simulink model "fanghua"  (R2022b)
settings: Solver=FixedStepDiscrete  StartTime=0.0  StopTime=10.0  FixedStep=0.01  RelTol=1e-3
undefined symbols (not defined in the file): R, sigbuilder_block
libraries: simulink x10
settings Model: Creator=YJR  LastModifiedBy=YJR

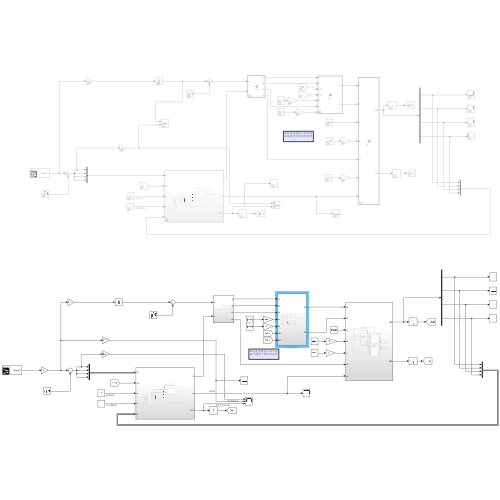
[thumbnail: Simulink's stored preview of the top-level diagram]
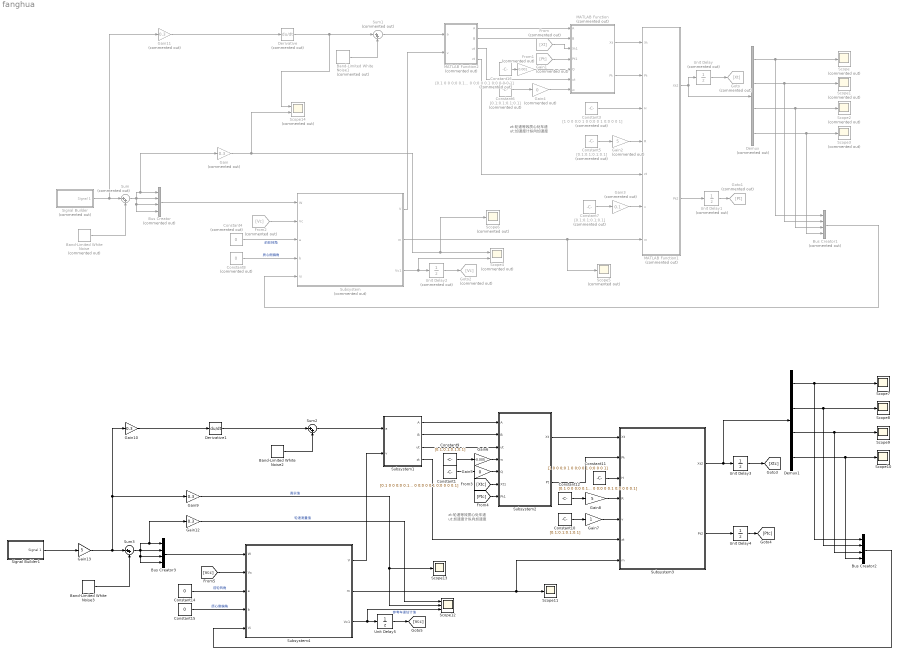
== system fanghua ==
  note: zt:轮速等效质心处车速
      | ut:加速度计纵向加速度
  note: zt:轮速等效质心处车速
      | ut:加速度计纵向加速度
  Band-Limited White Noise : simulink/Sources/Band-Limited White Noise  Commented=on  Cov=[0.05]  Ts=0.05  seed=[23341]
  Band-Limited White Noise1 : simulink/Sources/Band-Limited White Noise  Commented=on  Cov=[0.1]  Ts=0.1  seed=[23341]
  Band-Limited White Noise2 : simulink/Sources/Band-Limited White Noise  Cov=[0.1]  Ts=0.01  seed=[23341]
  Band-Limited White Noise3 : simulink/Sources/Band-Limited White Noise  Cov=[0.05]  Ts=0.01  seed=[23341]
  Bus Creator : BusCreator  Commented=on  Inputs=4
  Bus Creator1 : BusCreator  Commented=on  Inputs=4
  Bus Creator2 : BusCreator  Inputs=4
  Bus Creator3 : BusCreator  Inputs=4
  Constant1 : Constant  Value=[0.1 0 0 0;0 0.1 0 0;0 0 0.1 0;0 0 0 0.1]
  Constant10 : Constant  Value=[0.1;0.1;0.1;0.1]
  Constant11 : Constant  Value=[1 0 0 0;0 1 0 0;0 0 1 0;0 0 0 1]
  Constant12 : Constant  Value=[0.1 0 0 0;0 0.1 0 0;0 0 0.1 0;0 0 0 0.1]
  Constant14 : Constant  Value=0
  Constant15 : Constant  Value=0
  Constant16 : Constant  Commented=on  Value=[0.1 0 0 0;0 0.1 0 0;0 0 0.1 0;0 0 0 0.1]
  Constant3 : Constant  Commented=on  Value=[1 0 0 0;0 1 0 0;0 0 1 0;0 0 0 1]
  Constant4 : Constant  Commented=on  Value=0
  Constant5 : Constant  Commented=on  Value=[0.1;0.1;0.1;0.1]
  Constant6 : Constant  Commented=on  Value=[0.1;0.1;0.1;0.1]
  Constant7 : Constant  Commented=on  Value=[0.1;0.1;0.1;0.1]
  Constant8 : Constant  Commented=on  Value=0
  Constant9 : Constant  Value=[0.1;0.1;0.1;0.1]
  Demux : Demux  Commented=on
  Demux1 : Demux
  Derivative : Derivative  Commented=on
  Derivative1 : Derivative
  From : From  Commented=on  GotoTag=Xt
  From1 : From  Commented=on  GotoTag=Pt
  From2 : From  Commented=on  GotoTag=Vc
  Gain : Gain  Commented=on  Gain=0.3
  Gain1 : Gain  Commented=on  Gain=0.001
  Gain10 : Gain  Gain=0.3
  Gain11 : Gain  Commented=on  Gain=0.3
  Gain12 : Gain  Gain=0.3
  Gain13 : Gain  Gain=5
  Gain2 : Gain  Commented=on  Gain=5
  Gain3 : Gain  Commented=on  Gain=0.1
  Gain4 : Gain  Commented=on  Gain=0
  Gain5 : Gain  Gain=0
  Gain6 : Gain  Gain=-0.005
  Gain7 : Gain
  Gain8 : Gain  Gain=5
  Gain9 : Gain  Gain=0.3
  Goto : Goto  Commented=on  GotoTag=Xt
  Goto1 : Goto  Commented=on  GotoTag=Pt
  Goto2 : Goto  Commented=on  GotoTag=Vc
  MATLAB Function : MATLAB Function  Commented=on  TreatAsAtomicUnit=on
  MATLAB Function1 : MATLAB Function  Commented=on  TreatAsAtomicUnit=on
  MATLAB Function2 : MATLAB Function  Commented=on  TreatAsAtomicUnit=on
  Scope{,1..3,5..6} (6 alike) : Scope  Commented=on
  Scope{7..11,13} (6 alike) : Scope
  Scope12 : Scope  NumInputPorts=3
  Scope14 : Scope  Commented=on  NumInputPorts=2
  Scope4 : Scope  Commented=on  NumInputPorts=2
  Signal Builder : Subsystem  Tag=STV Subsys  Commented=on  LoadFcn=sigbuilder_block('load');  StartFcn=sigbuilder_block('start');  StopFcn=sigbuilder_block('stop');  ClipboardFcn=sigbuilder_block('clipboard');  mask(Sigbuilder block){tuvar=[0:10]}
      mask help: Simulink:masks:SigbuilderBlock_MD
      mask init:
      | if ~strcmp(get_param(bdroot(gcbh),'SimulationStatus'),'stopped') tuvar = sigbuilder_block('maskInit'); end
      settings: CopyFcn=sigbuilder_block('copy');  DeleteFcn=sigbuilder_block('delete');  ModelCloseFcn=sigbuilder_block('modelClose');  PreSaveFcn=sigbuilder_block('preSave');  PauseFcn=sigbuilder_block('pause');  ContinueFcn=sigbuilder_block('continue');  NameChangeFcn=sigbuilder_block('namechange');  OpenFcn=sigbuilder_block('open',[437.6 199.2 550.4 400 ]);  CloseFcn=sigbuilder_block('close');
      mask Display: plot(0, 0, 100, 100,[2, 2, 32, 32, 2], [68, 8, 8, 68, 68],[32, 2], [38, 38], [32, 19, 2],[53, 60, 44], [32, 17, 17, 2],[16, 16, 31, 31]);txt = getActiveGroup(gcbh);text(2, 100, txt,'verticalAlignment', 'top');
  Signal Builder1 : Subsystem  Tag=STV Subsys  LoadFcn=sigbuilder_block('load');  StartFcn=sigbuilder_block('start');  StopFcn=sigbuilder_block('stop');  ClipboardFcn=sigbuilder_block('clipboard');  mask(Sigbuilder block){tuvar=[0:10]}
      mask help: Simulink:masks:SigbuilderBlock_MD
      mask init:
      | if ~strcmp(get_param(bdroot(gcbh),'SimulationStatus'),'stopped') tuvar = sigbuilder_block('maskInit'); end
      settings: CopyFcn=sigbuilder_block('copy');  DeleteFcn=sigbuilder_block('delete');  ModelCloseFcn=sigbuilder_block('modelClose');  PreSaveFcn=sigbuilder_block('preSave');  PauseFcn=sigbuilder_block('pause');  ContinueFcn=sigbuilder_block('continue');  NameChangeFcn=sigbuilder_block('namechange');  OpenFcn=sigbuilder_block('open',[437.6 199.2 550.4 400 ]);  CloseFcn=sigbuilder_block('close');
      mask Display: plot(0, 0, 100, 100,[2, 2, 32, 32, 2], [68, 8, 8, 68, 68],[32, 2], [38, 38], [32, 19, 2],[53, 60, 44], [32, 17, 17, 2],[16, 16, 31, 31]);txt = getActiveGroup(gcbh);text(2, 100, txt,'verticalAlignment', 'top');
  Subsystem : Subsystem  Commented=on
  Subsystem1 : Subsystem
  Subsystem2 : Subsystem
  Subsystem3 : Subsystem
  Subsystem4 : Subsystem
  Sum : Sum  Commented=on  Inputs=|++
  Sum1 : Sum  Commented=on  Inputs=|++
  Sum2 : Sum  Inputs=|++
  Sum3 : Sum  Inputs=|++
  Unit Delay : UnitDelay  Commented=on  SampleTime=-1  HasFrameUpgradeWarning=on
  Unit Delay1 : UnitDelay  Commented=on  SampleTime=-1  HasFrameUpgradeWarning=on
  Unit Delay2 : UnitDelay  Commented=on  SampleTime=-1  HasFrameUpgradeWarning=on
  Unit Delay3 : UnitDelay  SampleTime=-1  HasFrameUpgradeWarning=on
  Unit Delay4 : UnitDelay  SampleTime=-1  HasFrameUpgradeWarning=on
  Unit Delay5 : UnitDelay  SampleTime=-1  HasFrameUpgradeWarning=on
  wires:
  MATLAB Function1/2(Pt2) -> Unit Delay1/1
  MATLAB Function/1(Xt) -> MATLAB Function1/1(Xt)
  MATLAB Function/2(Pt) -> MATLAB Function1/2(Pt)
  MATLAB Function2/1(A) -> MATLAB Function/1(A)
  MATLAB Function2/2(B) -> MATLAB Function/2(B)
  Constant16/1 -> Gain1/1
  Constant3/1 -> MATLAB Function1/3(H)
  MATLAB Function2/3(ut) -> MATLAB Function/6(ut)
  Demux/1 -> Bus Creator1/1, Scope/1
  Demux/2 -> Bus Creator1/2, Scope1/1
  Constant5/1 -> Gain2/1
  MATLAB Function2/4(zt) -> MATLAB Function1/5(zt)
  Constant6/1 -> Gain4/1
  From/1 -> MATLAB Function/3(Xt1)
  Unit Delay/1 -> Goto/1
  From1/1 -> MATLAB Function/4(Pt1)
  Unit Delay1/1 -> Goto1/1
  Constant7/1 -> Gain3/1
  Demux/3 -> Bus Creator1/3, Scope2/1
  Demux/4 -> Bus Creator1/4, Scope3/1
  Subsystem/2(m) -> Scope5/1, MATLAB Function1/7(m)
  Gain1/1 -> MATLAB Function/5(Q)
  Gain2/1 -> MATLAB Function1/4(R)
  Gain3/1 -> MATLAB Function1/6(v)
  Subsystem/1(V) -> MATLAB Function2/2(v)
  Subsystem/3(Vc1) -> Scope4/2, Unit Delay2/1
  From2/1 -> Subsystem/2(Vc)
  Unit Delay2/1 -> Goto2/1
  MATLAB Function1/1(Xt2) -> Unit Delay/1, Demux/1
  Bus Creator1/1 -> Subsystem/5(Vi)
  Constant4/1 -> Subsystem/3(a)  "前轮转角"
  Constant8/1 -> Subsystem/4(b)  "质心侧偏角"
  Bus Creator/1 -> Subsystem/1(W)
  Sum/1 -> Gain/1, Bus Creator/1, Bus Creator/2, Bus Creator/3, Bus Creator/4
  Gain/1 -> Scope14/2, Scope6/1, Scope4/1
  Band-Limited White Noise/1 -> Sum/2
  Sum1/1 -> MATLAB Function2/1(a)
  Gain4/1 -> MATLAB Function/7(w)
  Derivative/1 -> Scope14/1, Sum1/1
  Band-Limited White Noise1/1 -> Sum1/2
  Subsystem1/1(A) -> Subsystem2/1(A)
  Subsystem1/2(B) -> Subsystem2/2(B)
  Subsystem1/3(ut) -> Subsystem2/3(ut)
  Gain5/1 -> Subsystem2/5(Q)
  Constant1/1 -> Gain5/1
  Constant9/1 -> Gain6/1
  Gain6/1 -> Subsystem2/4(w)
  [Xtc] -> Subsystem2/6(Xt1)
  [Ptc] -> Subsystem2/7(Pt1)
  Constant10/1 -> Gain7/1
  Gain7/1 -> Subsystem3/5(v)
  Subsystem1/4(zt) -> Subsystem3/6(zt)
  Subsystem2/1(Xt) -> Subsystem3/1(Xt)
  Subsystem2/2(Pt) -> Subsystem3/2(Pt)
  Constant11/1 -> Subsystem3/3(H)
  Constant12/1 -> Gain8/1
  Gain8/1 -> Subsystem3/4(R)
  Subsystem3/1(Xt2) -> Demux1/1, Unit Delay3/1
  Unit Delay3/1 -> [Xtc]
  Unit Delay4/1 -> [Ptc]
  Subsystem3/2(Pt2) -> Unit Delay4/1
  Band-Limited White Noise2/1 -> Sum2/2
  Derivative1/1 -> Sum2/1
  Sum2/1 -> Subsystem1/1(a)
  Demux1/4 -> Scope10/1, Bus Creator2/4
  Demux1/3 -> Scope9/1, Bus Creator2/3
  Demux1/2 -> Scope8/1, Bus Creator2/2
  Demux1/1 -> Scope7/1, Bus Creator2/1
  Band-Limited White Noise3/1 -> Sum3/2
  Gain9/1 -> Scope12/2, Scope13/1  "真实值"
  Sum3/1 -> Bus Creator3/4, Bus Creator3/3, Bus Creator3/2, Gain12/1, Bus Creator3/1
  Bus Creator3/1 -> Subsystem4/1(W)
  Constant15/1 -> Subsystem4/4(b)  "质心侧偏角"
  Constant14/1 -> Subsystem4/3(a)  "前轮转角"
  Bus Creator2/1 -> Subsystem4/5(Vi)
  Signal Builder1/1(Signal 1) -> Gain13/1
  Unit Delay5/1 -> [Vcc]
  [Vcc] -> Subsystem4/2(Vc)
  Subsystem4/3(Vc1) -> Scope12/3, Unit Delay5/1  "参考车速估计值"
  Subsystem4/1(V) -> Subsystem1/2(v)
  Subsystem4/2(m) -> Scope11/1, Subsystem3/7(m)
  Signal Builder/1(Signal 1) -> Gain11/1, Sum/1
  Gain10/1 -> Derivative1/1
  Gain11/1 -> Derivative/1
  Gain12/1 -> Scope12/1  "轮速测量值"
  Gain13/1 -> Gain9/1, Gain10/1, Sum3/1

== system fanghua/Signal Builder ==
  Demux : Demux  Tag=STV Demux  Outputs=1
      settings: DisplayOption=none
  FromWs : FromWorkspace  Tag=STV FromWs  VariableName=tuvar
      SigBuilderData=|
      | common.afterFinalStr = 'Extrapolate'
      | common.sampleTime = 0
      | dataSet.timeRange = [0 10]
      | dataSet.name = 'Group 1'
      | sbobj.Groups.Name = 'Group 1'
      | sbobj.Groups.Signals.Name = 'Signal 1'
      | sbobj.Groups.Signals.XData = [0 3 4 6 8 10]
      | sbobj.Groups.Signals.YData = [0 6.8 30 26.4 0 0]
  Signal 1 : Outport  Tag=STV Outport
  wires:
  FromWs/1 -> Demux/1
  Demux/1 -> Signal 1/1

== system fanghua/Signal Builder1 ==
  Demux : Demux  Tag=STV Demux  Outputs=1
      settings: DisplayOption=none
  FromWs : FromWorkspace  Tag=STV FromWs  VariableName=tuvar
      SigBuilderData=|
      | common.afterFinalStr = 'Extrapolate'
      | common.sampleTime = 0
      | dataSet.timeRange = [0 10]
      | dataSet.name = 'Group 1'
      | sbobj.Groups.Name = 'Group 1'
      | sbobj.Groups.Signals.Name = 'Signal 1'
      | sbobj.Groups.Signals.XData = [0 3 4 6 8 10]
      | sbobj.Groups.Signals.YData = [0 6.8 30 22 36 0]
  Signal 1 : Outport  Tag=STV Outport
  wires:
  Demux/1 -> Signal 1/1
  FromWs/1 -> Demux/1

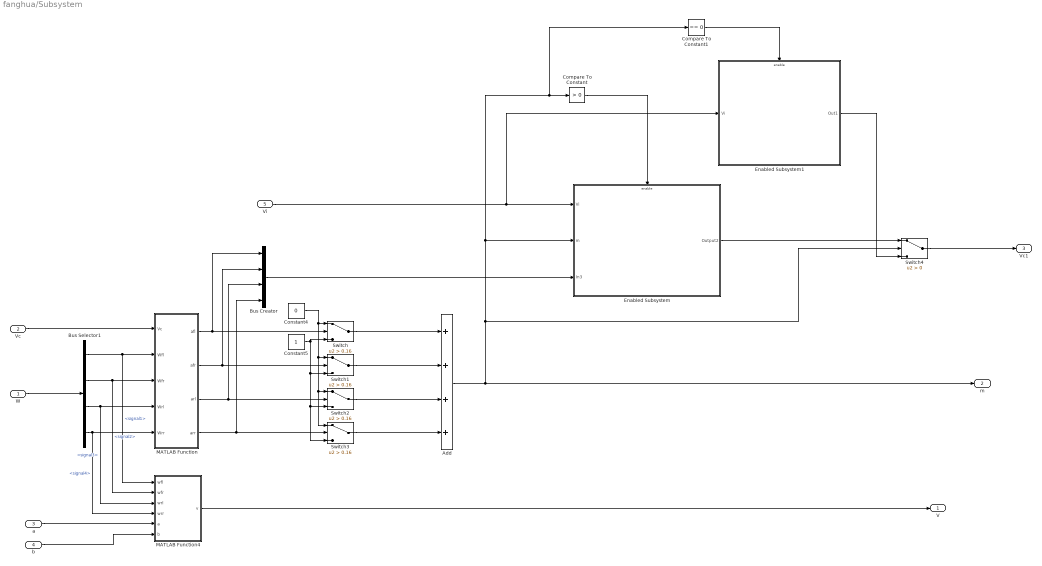
== system fanghua/Subsystem ==
  W : Inport
  Vc : Inport  Port=2
  a : Inport  Port=3
  b : Inport  Port=4
  Vi : Inport  Port=5
  Add : Sum  Inputs=++++
  Bus Creator : BusCreator  Inputs=4
  Bus Selector1 : BusSelector  OutputSignals=signal1,signal2,signal3,signal4
  Compare To Constant : simulink/Logic and Bit Operations/Compare To Constant  relop=>  const=0  OutDataTypeStr=boolean
  Compare To Constant1 : simulink/Logic and Bit Operations/Compare To Constant  relop===  const=0  OutDataTypeStr=boolean
  Constant4 : Constant  Value=0
  Constant5 : Constant
  Enabled Subsystem : Subsystem  TreatAsAtomicUnit=on
  Enabled Subsystem1 : Subsystem  TreatAsAtomicUnit=on
  MATLAB Function : MATLAB Function  TreatAsAtomicUnit=on
  MATLAB Function4 : MATLAB Function  TreatAsAtomicUnit=on
  Switch{,1..3} (4 alike) : Switch  Criteria=u2 > Threshold  Threshold=0.16  SaturateOnIntegerOverflow=off  InputSameDT=off
  Switch4 : Switch  Criteria=u2 > Threshold  SaturateOnIntegerOverflow=off  InputSameDT=off
  V : Outport
  m : Outport  Port=2
  Vc1 : Outport  Port=3
  wires:
  Constant5/1 -> Switch3/3, Switch2/3, Switch1/3, Switch/3
  Constant4/1 -> Switch3/1, Switch2/1, Switch1/1, Switch/1
  Add/1 -> Switch4/2, Enabled Subsystem/2(m), Compare To Constant1/1, Compare To Constant/1, m/1
  Bus Selector1/1 -> MATLAB Function4/1(wfl), MATLAB Function/2(Wfl)  "<signal1>"
  Bus Selector1/2 -> MATLAB Function4/2(wfr), MATLAB Function/3(Wfr)  "<signal2>"
  Bus Selector1/3 -> MATLAB Function4/3(wrl), MATLAB Function/4(Wrl)  "<signal3>"
  Bus Selector1/4 -> MATLAB Function4/4(wrr), MATLAB Function/5(Wrr)  "<signal4>"
  W/1 -> Bus Selector1/1
  MATLAB Function/1(afl) -> Bus Creator/1, Switch/2
  MATLAB Function/2(afr) -> Bus Creator/2, Switch1/2
  MATLAB Function/3(arl) -> Bus Creator/3, Switch2/2
  MATLAB Function/4(arr) -> Bus Creator/4, Switch3/2
  Vc/1 -> MATLAB Function/1(Vc)
  MATLAB Function4/1(v) -> V/1
  Switch/1 -> Add/1
  Switch3/1 -> Add/4
  Switch2/1 -> Add/3
  Switch1/1 -> Add/2
  a/1 -> MATLAB Function4/5(a)
  b/1 -> MATLAB Function4/6(b)
  Vi/1 -> Enabled Subsystem1/1(Vi), Enabled Subsystem/1(Vi)
  Compare To Constant/1 -> Enabled Subsystem/Enable
  Bus Creator/1 -> Enabled Subsystem/3(In3)
  Compare To Constant1/1 -> Enabled Subsystem1/Enable
  Enabled Subsystem/1(Output2) -> Switch4/1
  Enabled Subsystem1/1(Out1) -> Switch4/3
  Switch4/1 -> Vc1/1

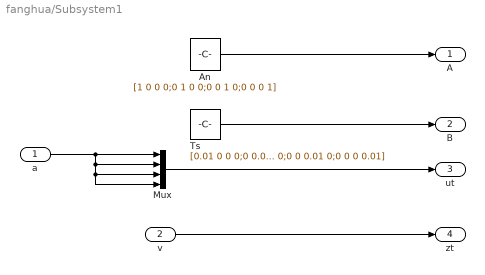
== system fanghua/Subsystem1 ==
  a : Inport
  v : Inport  Port=2
  An : Constant  Value=[1 0 0 0;0 1 0 0;0 0 1 0;0 0 0 1]
  Mux : Mux
  Ts : Constant  Value=[0.01 0 0 0;0 0.01 0 0;0 0 0.01 0;0 0 0 0.01]
  A : Outport
  B : Outport  Port=2
  ut : Outport  Port=3
  zt : Outport  Port=4
  wires:
  v/1 -> zt/1
  Mux/1 -> ut/1
  a/1 -> Mux/1, Mux/4, Mux/3, Mux/2
  An/1 -> A/1
  Ts/1 -> B/1

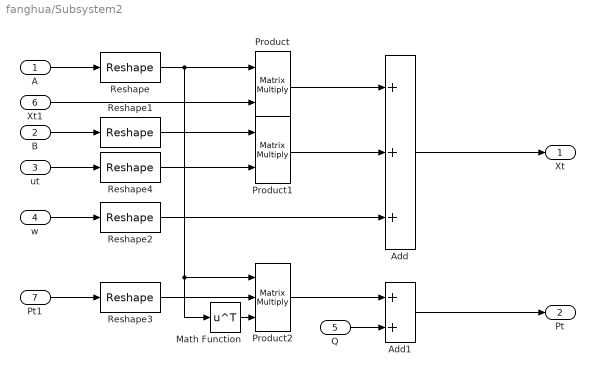
== system fanghua/Subsystem2 ==
  A : Inport
  B : Inport  Port=2
  ut : Inport  Port=3
  w : Inport  Port=4
  Q : Inport  Port=5
  Xt1 : Inport  Port=6
  Pt1 : Inport  Port=7
  Add : Sum  Inputs=+++
  Add1 : Sum
  Math Function : Math  Operator=transpose
  Product : Product  Multiplication=Matrix(*)
  Product1 : Product  Multiplication=Matrix(*)
  Product2 : Product  Inputs=3  Multiplication=Matrix(*)
  Reshape : Reshape  OutputDimensionality=Customize  OutputDimensions=[4,4]
  Reshape1 : Reshape  OutputDimensionality=Customize  OutputDimensions=[4,4]
  Reshape2 : Reshape  OutputDimensionality=Customize  OutputDimensions=[4,1]
  Reshape3 : Reshape  OutputDimensionality=Customize  OutputDimensions=[4,4]
  Reshape4 : Reshape  OutputDimensionality=Customize  OutputDimensions=[4,1]
  Xt : Outport
  Pt : Outport  Port=2
  wires:
  A/1 -> Reshape/1
  B/1 -> Reshape1/1
  Reshape/1 -> Math Function/1, Product2/1, Product/1
  Product/1 -> Add/1
  Xt1/1 -> Product/2
  Reshape1/1 -> Product1/1
  ut/1 -> Reshape4/1
  w/1 -> Reshape2/1
  Product1/1 -> Add/2
  Reshape2/1 -> Add/3
  Add/1 -> Xt/1
  Pt1/1 -> Reshape3/1
  Math Function/1 -> Product2/3
  Product2/1 -> Add1/1
  Q/1 -> Add1/2
  Add1/1 -> Pt/1
  Reshape3/1 -> Product2/2
  Reshape4/1 -> Product1/2

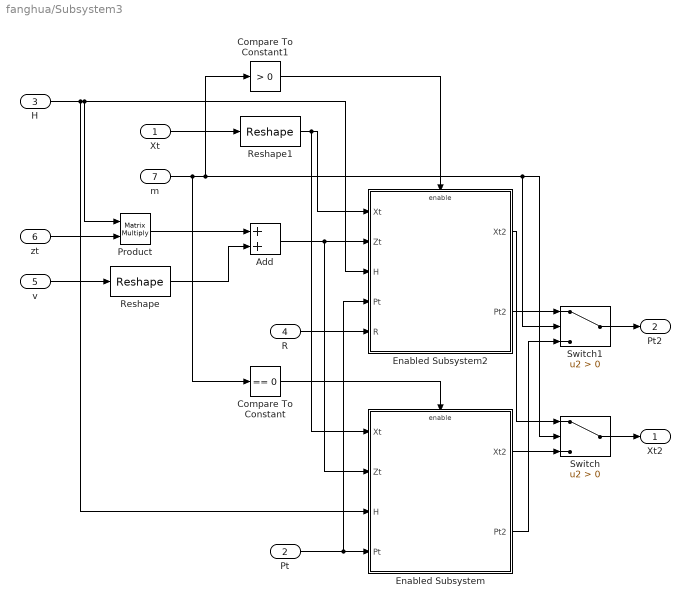
== system fanghua/Subsystem3 ==
  Xt : Inport
  Pt : Inport  Port=2
  H : Inport  Port=3
  R : Inport  Port=4
  v : Inport  Port=5
  zt : Inport  Port=6
  m : Inport  Port=7
  Add : Sum
  Compare To Constant : simulink/Logic and Bit Operations/Compare To Constant  relop===  const=0  OutDataTypeStr=boolean
  Compare To Constant1 : simulink/Logic and Bit Operations/Compare To Constant  relop=>  const=0  OutDataTypeStr=boolean
  Enabled Subsystem : Subsystem  TreatAsAtomicUnit=on
  Enabled Subsystem2 : Subsystem  TreatAsAtomicUnit=on
  Product : Product  Multiplication=Matrix(*)
  Reshape : Reshape  OutputDimensionality=Customize  OutputDimensions=[4,1]
  Reshape1 : Reshape  OutputDimensionality=Customize  OutputDimensions=[4,1]
  Switch : Switch  Criteria=u2 > Threshold  SaturateOnIntegerOverflow=off  InputSameDT=off
  Switch1 : Switch  Criteria=u2 > Threshold  SaturateOnIntegerOverflow=off  InputSameDT=off
  Xt2 : Outport
  Pt2 : Outport  Port=2
  wires:
  H/1 -> Enabled Subsystem2/3(H), Product/1, Enabled Subsystem/3(H)
  Switch/1 -> Xt2/1
  Compare To Constant1/1 -> Enabled Subsystem2/Enable
  zt/1 -> Product/2
  Enabled Subsystem/1(Xt2) -> Switch/3
  Reshape/1 -> Add/2
  Compare To Constant/1 -> Enabled Subsystem/Enable
  v/1 -> Reshape/1
  Product/1 -> Add/1
  m/1 -> Switch1/2, Switch/2, Compare To Constant1/1, Compare To Constant/1
  Xt/1 -> Reshape1/1
  Reshape1/1 -> Enabled Subsystem2/1(Xt), Enabled Subsystem/1(Xt)
  Add/1 -> Enabled Subsystem/2(Zt), Enabled Subsystem2/2(Zt)
  R/1 -> Enabled Subsystem2/5(R)
  Pt/1 -> Enabled Subsystem/4(Pt), Enabled Subsystem2/4(Pt)
  Enabled Subsystem2/1(Xt2) -> Switch/1
  Enabled Subsystem2/2(Pt2) -> Switch1/1
  Enabled Subsystem/2(Pt2) -> Switch1/3
  Switch1/1 -> Pt2/1

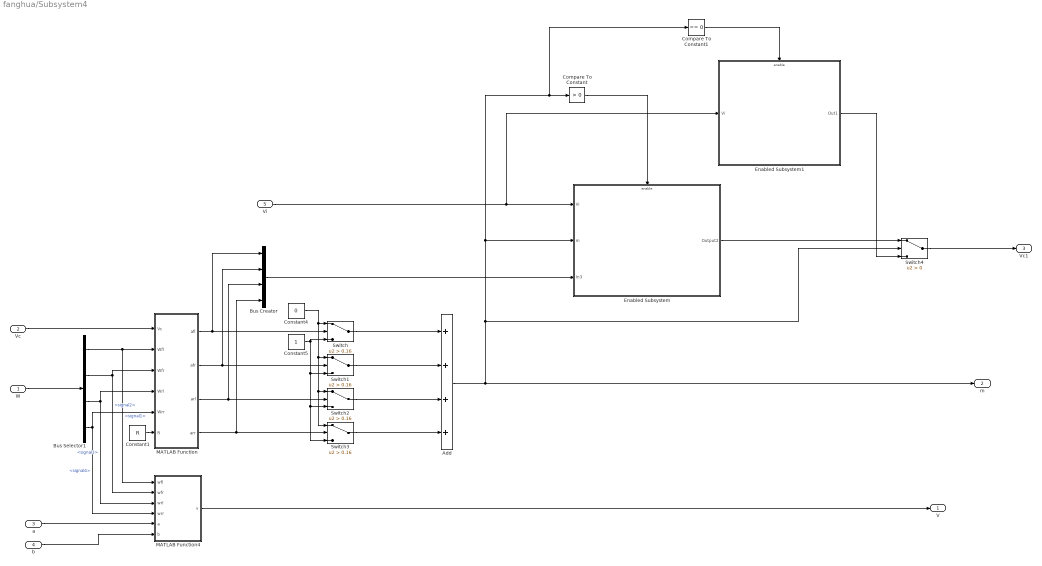
== system fanghua/Subsystem4 ==
  W : Inport
  Vc : Inport  Port=2
  a : Inport  Port=3
  b : Inport  Port=4
  Vi : Inport  Port=5
  Add : Sum  Inputs=++++
  Bus Creator : BusCreator  Inputs=4
  Bus Selector1 : BusSelector  OutputSignals=signal1,signal2,signal3,signal4
  Compare To Constant : simulink/Logic and Bit Operations/Compare To Constant  relop=>  const=0  OutDataTypeStr=boolean
  Compare To Constant1 : simulink/Logic and Bit Operations/Compare To Constant  relop===  const=0  OutDataTypeStr=boolean
  Constant1 : Constant  Value=R
  Constant4 : Constant  Value=0
  Constant5 : Constant
  Enabled Subsystem : Subsystem  TreatAsAtomicUnit=on
  Enabled Subsystem1 : Subsystem  TreatAsAtomicUnit=on
  MATLAB Function : MATLAB Function  TreatAsAtomicUnit=on
  MATLAB Function4 : MATLAB Function  TreatAsAtomicUnit=on
  Switch{,1..3} (4 alike) : Switch  Criteria=u2 > Threshold  Threshold=0.16  SaturateOnIntegerOverflow=off  InputSameDT=off
  Switch4 : Switch  Criteria=u2 > Threshold  SaturateOnIntegerOverflow=off  InputSameDT=off
  V : Outport
  m : Outport  Port=2
  Vc1 : Outport  Port=3
  wires:
  Switch4/1 -> Vc1/1
  Enabled Subsystem1/1(Out1) -> Switch4/3
  Enabled Subsystem/1(Output2) -> Switch4/1
  Compare To Constant1/1 -> Enabled Subsystem1/Enable
  Bus Creator/1 -> Enabled Subsystem/3(In3)
  Compare To Constant/1 -> Enabled Subsystem/Enable
  Vi/1 -> Enabled Subsystem/1(Vi), Enabled Subsystem1/1(Vi)
  b/1 -> MATLAB Function4/6(b)
  a/1 -> MATLAB Function4/5(a)
  Switch1/1 -> Add/2
  Switch2/1 -> Add/3
  Switch3/1 -> Add/4
  Switch/1 -> Add/1
  MATLAB Function4/1(v) -> V/1
  Vc/1 -> MATLAB Function/1(Vc)
  MATLAB Function/4(arr) -> Switch3/2, Bus Creator/4
  MATLAB Function/3(arl) -> Switch2/2, Bus Creator/3
  MATLAB Function/2(afr) -> Switch1/2, Bus Creator/2
  MATLAB Function/1(afl) -> Switch/2, Bus Creator/1
  W/1 -> Bus Selector1/1
  Bus Selector1/4 -> MATLAB Function4/4(wrr), MATLAB Function/5(Wrr)  "<signal4>"
  Bus Selector1/3 -> MATLAB Function4/3(wrl), MATLAB Function/4(Wrl)  "<signal3>"
  Bus Selector1/2 -> MATLAB Function4/2(wfr), MATLAB Function/3(Wfr)  "<signal2>"
  Bus Selector1/1 -> MATLAB Function4/1(wfl), MATLAB Function/2(Wfl)  "<signal1>"
  Add/1 -> m/1, Compare To Constant/1, Compare To Constant1/1, Enabled Subsystem/2(m), Switch4/2
  Constant4/1 -> Switch/1, Switch1/1, Switch2/1, Switch3/1
  Constant5/1 -> Switch/3, Switch1/3, Switch2/3, Switch3/3
  Constant1/1 -> MATLAB Function/6(R)

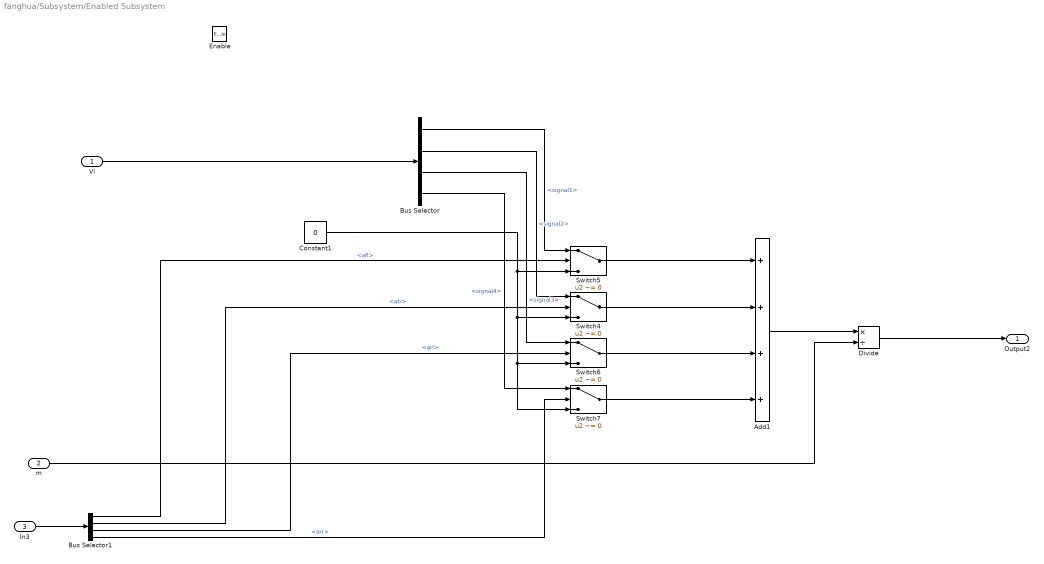
== system fanghua/Subsystem/Enabled Subsystem ==
  Vi : Inport
  m : Inport  Port=2
  In3 : Inport  Port=3
  Enable : EnablePort
  Add1 : Sum  Inputs=++++
  Bus Selector : BusSelector  OutputSignals=signal1,signal2,signal3,signal4
  Bus Selector1 : BusSelector  OutputSignals=afl,afr,arl,arr
  Constant1 : Constant  Value=0
  Divide : Product  Inputs=*/
  Switch{4..7} (4 alike) : Switch  Criteria=u2 ~= 0  Threshold=1  SaturateOnIntegerOverflow=off  InputSameDT=off
  Output2 : Outport
  wires:
  Bus Selector1/3 -> Switch6/2  "<arl>"
  Switch4/1 -> Add1/2
  Bus Selector1/2 -> Switch4/2  "<afr>"
  Bus Selector/3 -> Switch6/1  "<signal3>"
  Bus Selector/2 -> Switch4/1  "<signal2>"
  Constant1/1 -> Switch6/3, Switch7/3, Switch4/3, Switch5/3
  Bus Selector/1 -> Switch5/1  "<signal1>"
  m/1 -> Divide/2
  Bus Selector1/4 -> Switch7/2  "<arr>"
  Switch7/1 -> Add1/4
  Vi/1 -> Bus Selector/1
  Bus Selector/4 -> Switch7/1  "<signal4>"
  Switch6/1 -> Add1/3
  Add1/1 -> Divide/1
  Divide/1 -> Output2/1
  Switch5/1 -> Add1/1
  Bus Selector1/1 -> Switch5/2  "<afl>"
  In3/1 -> Bus Selector1/1

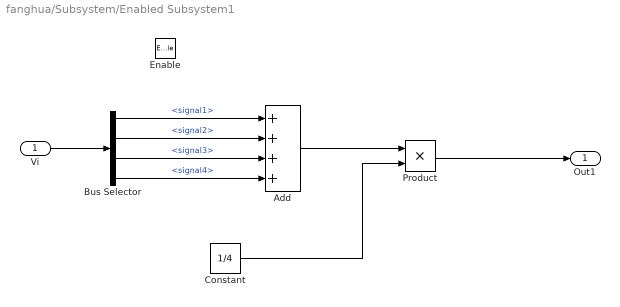
== system fanghua/Subsystem/Enabled Subsystem1 ==
  Vi : Inport
  Enable : EnablePort
  Add : Sum  Inputs=++++
  Bus Selector : BusSelector  OutputSignals=signal1,signal2,signal3,signal4
  Constant : Constant  Value=1/4
  Product : Product
  Out1 : Outport
  wires:
  Vi/1 -> Bus Selector/1
  Bus Selector/1 -> Add/1  "<signal1>"
  Bus Selector/3 -> Add/3  "<signal3>"
  Bus Selector/2 -> Add/2  "<signal2>"
  Bus Selector/4 -> Add/4  "<signal4>"
  Constant/1 -> Product/2
  Add/1 -> Product/1
  Product/1 -> Out1/1

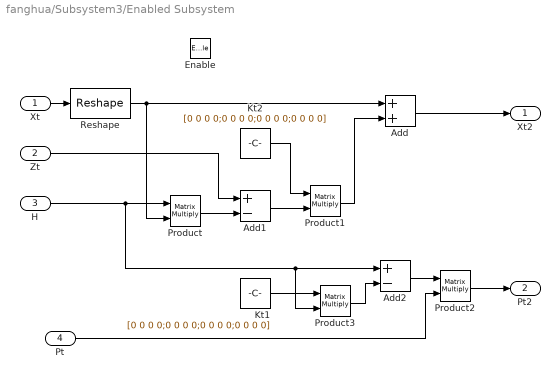
== system fanghua/Subsystem3/Enabled Subsystem ==
  Xt : Inport
  Zt : Inport  Port=2
  H : Inport  Port=3
  Pt : Inport  Port=4
  Enable : EnablePort
  Add : Sum
  Add1 : Sum  Inputs=+-
  Add2 : Sum  Inputs=+-
  Kt1 : Constant  Value=[0 0 0 0;0 0 0 0;0 0 0 0;0 0 0 0]
  Kt2 : Constant  Value=[0 0 0 0;0 0 0 0;0 0 0 0;0 0 0 0]
  Product{,1..3} (4 alike) : Product  Multiplication=Matrix(*)
  Reshape : Reshape  OutputDimensionality=Customize  OutputDimensions=[4,1]
  Xt2 : Outport
  Pt2 : Outport  Port=2
  wires:
  Xt/1 -> Reshape/1
  Add/1 -> Xt2/1
  Product/1 -> Add1/2
  Zt/1 -> Add1/1
  Add1/1 -> Product1/2
  Product1/1 -> Add/2
  H/1 -> Product3/2, Add2/1, Product/1
  Product3/1 -> Add2/2
  Add2/1 -> Product2/1
  Pt/1 -> Product2/2
  Product2/1 -> Pt2/1
  Kt1/1 -> Product3/1
  Reshape/1 -> Product/2, Add/1
  Kt2/1 -> Product1/1

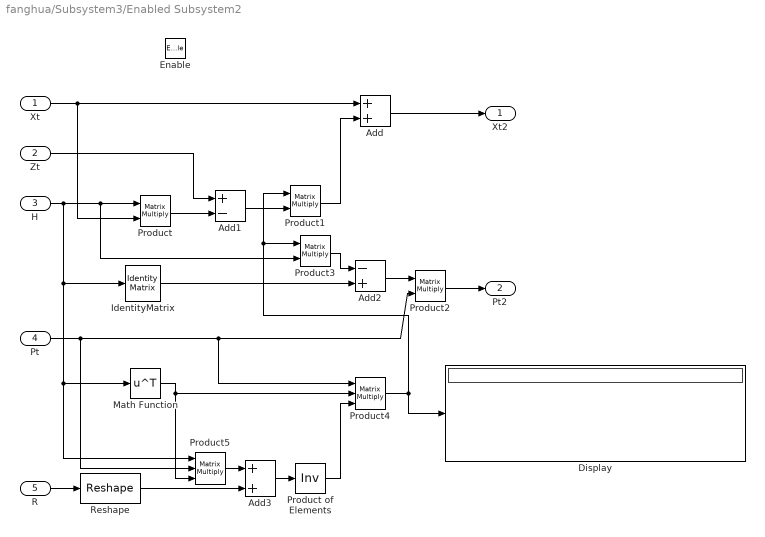
== system fanghua/Subsystem3/Enabled Subsystem2 ==
  Xt : Inport
  Zt : Inport  Port=2
  H : Inport  Port=3
  Pt : Inport  Port=4
  R : Inport  Port=5
  Enable : EnablePort
  Add : Sum
  Add1 : Sum  Inputs=+-
  Add2 : Sum  Inputs=-+
  Add3 : Sum
  Display : Display
  IdentityMatrix : IdentityMatrix  InheritOutputPortAttributes=on
  Math Function : Math  Operator=transpose
  Product{,1..3} (4 alike) : Product  Multiplication=Matrix(*)
  Product of Elements : Product  Inputs=/  Multiplication=Matrix(*)
  Product4 : Product  Inputs=3  Multiplication=Matrix(*)
  Product5 : Product  Inputs=3  Multiplication=Matrix(*)
  Reshape : Reshape  OutputDimensionality=Customize  OutputDimensions=[4,4]
  Xt2 : Outport
  Pt2 : Outport  Port=2
  wires:
  Product2/1 -> Pt2/1
  Pt/1 -> Product5/2, Product4/1, Product2/2
  Add2/1 -> Product2/1
  Product3/1 -> Add2/1
  IdentityMatrix/1 -> Add2/2
  Product1/1 -> Add/2
  Product4/1 -> Product1/1, Product3/1, Display/1
  Add1/1 -> Product1/2
  Zt/1 -> Add1/1
  Product/1 -> Add1/2
  H/1 -> Product/1, Product3/2, Product5/1, Math Function/1, IdentityMatrix/1
  Add/1 -> Xt2/1
  Xt/1 -> Add/1, Product/2
  Math Function/1 -> Product5/3, Product4/2
  Product5/1 -> Add3/1
  R/1 -> Reshape/1
  Add3/1 -> Product of Elements/1
  Product of Elements/1 -> Product4/3
  Reshape/1 -> Add3/2

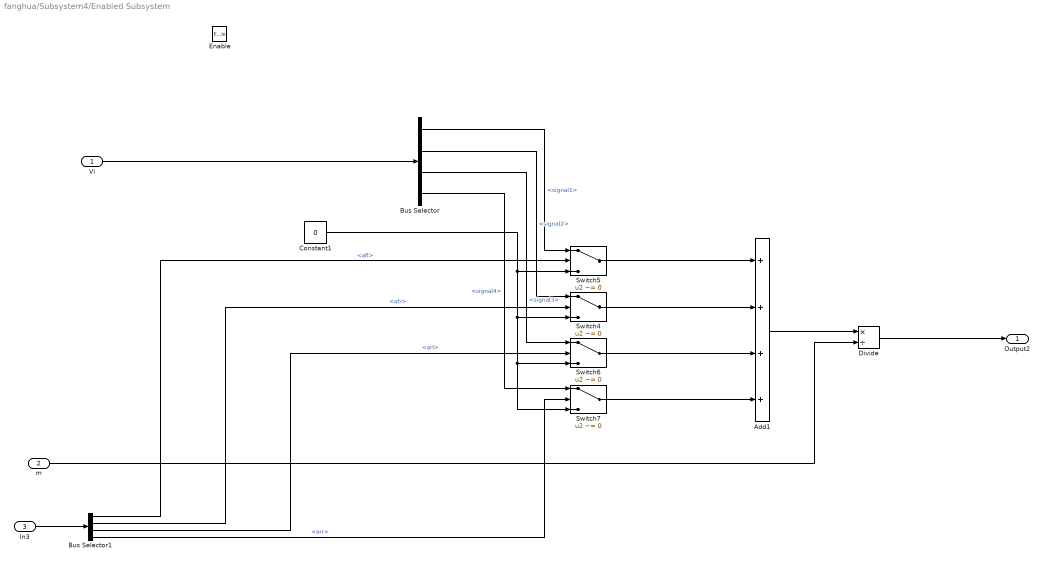
== system fanghua/Subsystem4/Enabled Subsystem ==
  Vi : Inport
  m : Inport  Port=2
  In3 : Inport  Port=3
  Enable : EnablePort
  Add1 : Sum  Inputs=++++
  Bus Selector : BusSelector  OutputSignals=signal1,signal2,signal3,signal4
  Bus Selector1 : BusSelector  OutputSignals=afl,afr,arl,arr
  Constant1 : Constant  Value=0
  Divide : Product  Inputs=*/
  Switch{4..7} (4 alike) : Switch  Criteria=u2 ~= 0  Threshold=1  SaturateOnIntegerOverflow=off  InputSameDT=off
  Output2 : Outport
  wires:
  In3/1 -> Bus Selector1/1
  Bus Selector1/1 -> Switch5/2  "<afl>"
  Switch5/1 -> Add1/1
  Divide/1 -> Output2/1
  Add1/1 -> Divide/1
  Switch6/1 -> Add1/3
  Bus Selector/4 -> Switch7/1  "<signal4>"
  Vi/1 -> Bus Selector/1
  Switch7/1 -> Add1/4
  Bus Selector1/4 -> Switch7/2  "<arr>"
  m/1 -> Divide/2
  Bus Selector/1 -> Switch5/1  "<signal1>"
  Constant1/1 -> Switch5/3, Switch4/3, Switch7/3, Switch6/3
  Bus Selector/2 -> Switch4/1  "<signal2>"
  Bus Selector/3 -> Switch6/1  "<signal3>"
  Bus Selector1/2 -> Switch4/2  "<afr>"
  Switch4/1 -> Add1/2
  Bus Selector1/3 -> Switch6/2  "<arl>"

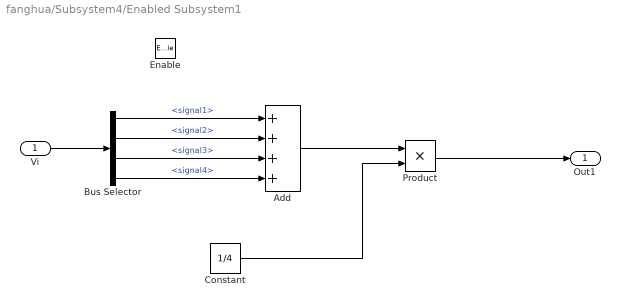
== system fanghua/Subsystem4/Enabled Subsystem1 ==
  Vi : Inport
  Enable : EnablePort
  Add : Sum  Inputs=++++
  Bus Selector : BusSelector  OutputSignals=signal1,signal2,signal3,signal4
  Constant : Constant  Value=1/4
  Product : Product
  Out1 : Outport
  wires:
  Product/1 -> Out1/1
  Add/1 -> Product/1
  Constant/1 -> Product/2
  Bus Selector/4 -> Add/4  "<signal4>"
  Bus Selector/2 -> Add/2  "<signal2>"
  Bus Selector/3 -> Add/3  "<signal3>"
  Bus Selector/1 -> Add/1  "<signal1>"
  Vi/1 -> Bus Selector/1

== matlab function fanghua/MATLAB Function1 ==
  data: Xt2 output; Xt input; Pt2 output; Pt input; H input; R input; zt input; v input; m input size=1
function [Xt2,Pt2] = fcn(Xt,Pt,H,R,zt,v,m)
Zt = H*zt+v;

if m == 0
    Kt = 0;
    Xt2 = Xt+Kt*(Zt-H*Xt);
    Pt2 = (eye(size(H))-Kt*H)*Pt;
else
    Kt = Pt*H'*(inv(H*Pt*H'+R));
    Xt2 = Xt+Kt*(Zt-H*Xt);
    Pt2 = (eye(size(H))-Kt*H)*Pt;
end



%v观测噪声
%H观测矩阵

== matlab function fanghua/MATLAB Function ==
  data: A input; Xt output size=[4,1]; B input; Pt output; Xt1 input size=[4,1]; Pt1 input size=[4,4]; Q input; ut input; w input
function [Xt,Pt] = fcn(A,B,Xt1,Pt1,Q,ut,w)

Xt = A*Xt1+B*ut+w;
Pt = A*Pt1*A'+Q;
%A系统矩阵
%w过程噪声
%P协方差矩阵
%Q过程噪声
%B控制矩阵

== matlab function fanghua/MATLAB Function2 ==
  data: A output; B output; ut output; a input; zt output; v input
function [A,B,ut,zt] = fcn(a,v)
A = [1 0 0 0;0 1 0 0;0 0 1 0;0 0 0 1];
B = [0.01 0 0 0;0 0.01 0 0;0 0 0.01 0;0 0 0 0.01];%Ts
ut = [a;a;a;a];
zt = v;

== matlab function fanghua/Subsystem4/MATLAB Function ==
  data: Vc input; afl output; Wfl input; Wfr input; Wrl input; Wrr input; afr output; arl output; arr output; R input
function [afl,afr,arl,arr] = fcn(Vc,Wfl,Wfr,Wrl,Wrr,R)
%轮胎半径
afl = abs((Wfl*R-Vc)/Wfl*R);
afr = abs((Wfr*R-Vc)/Wfr*R);
arl = abs((Wrl*R-Vc)/Wrl*R);
arr = abs((Wrr*R-Vc)/Wrr*R);

== matlab function fanghua/Subsystem/MATLAB Function ==
  data: Vc input; afl output; Wfl input; Wfr input; Wrl input; Wrr input; afr output; arl output; arr output
function [afl,afr,arl,arr] = fcn(Vc,Wfl,Wfr,Wrl,Wrr)
R = 0.3;%轮胎半径
afl = abs((Wfl*R-Vc)/Wfl*R);
afr = abs((Wfr*R-Vc)/Wfr*R);
arl = abs((Wrl*R-Vc)/Wrl*R);
arr = abs((Wrr*R-Vc)/Wrr*R);

== matlab function fanghua/Subsystem/MATLAB Function4 ==
  data: wfl input; v output size=[4,1]; wfr input; wrl input; wrr input; a input; b input
function v = fcn(wfl,wfr,wrl,wrr,a,b)
R = 0.3;%轮胎半径
lfw = 0.6;%前轮距
lrw = 0.6;%后轮距
lf = 0.8;%质心到前轴距离
lr = 0.8;%质心到后轴的距离
y = 1;
%a%前轮转角（二轮模型）
%b%质心侧偏角（二轮模型）
v = [(wfl*R+y*(lfw/2-lf*b))*cos(a-b);(wfr*R-y*(lfw/2-lf*b))*cos(a-b);(wrl*R+y*(lrw/2-lr*b))*cos(b);(wrr*R-y*(lrw/2-lr*b))*cos(b)];

== matlab function fanghua/Subsystem4/MATLAB Function4 ==
  data: wfl input; v output size=[4,1]; wfr input; wrl input; wrr input; a input; b input
function v = fcn(wfl,wfr,wrl,wrr,a,b)
R = 0.3;%轮胎半径
lfw = 0.6;%前轮距
lrw = 0.6;%后轮距
lf = 0.8;%质心到前轴距离
lr = 0.8;%质心到后轴的距离
y = 1;
%a%前轮转角（二轮模型）
%b%质心侧偏角（二轮模型）
v = [(wfl*R+y*(lfw/2-lf*b))*cos(a-b);(wfr*R-y*(lfw/2-lf*b))*cos(a-b);(wrl*R+y*(lrw/2-lr*b))*cos(b);(wrr*R-y*(lrw/2-lr*b))*cos(b)];
